simulink subsystem "decoder_8b10b"  (R2022b)
settings: Solver=VariableStepAuto  StartTime=0.0  StopTime=10.0  RelTol=1e-3
settings Model: Creator=Ali-Laptop  LastModifiedBy=Ali-Laptop

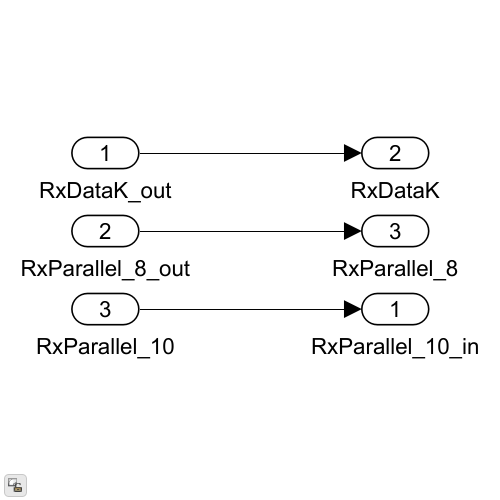
[thumbnail: Simulink's stored preview of the top-level diagram]
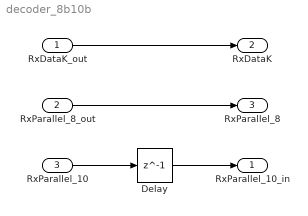
== system decoder_8b10b ==
  RxDataK_out : Inport
  RxParallel_8_out : Inport  Port=2
  RxParallel_10 : Inport  Port=3
  Delay : Delay  DelayLength=1
  RxParallel_10_in : Outport
  RxDataK : Outport  Port=2
  RxParallel_8 : Outport  Port=3
  wires:
  RxParallel_10/1 -> Delay/1
  RxDataK_out/1 -> RxDataK/1
  RxParallel_8_out/1 -> RxParallel_8/1
  Delay/1 -> RxParallel_10_in/1
